simulink model "qdrdacsim"  (R2012b)
(part 2 of 52)

  zero_bool_3 : xbsIndex_r4/Constant  const=1  gui_display_data_type=Boolean  arith_type=Boolean  n_bits=36  bin_pt=0  preci_type=Single  exp_width=8  frac_width=24  explicit_period=on  period=1  equ=P=C  opselect=C  inp2=PCIN>>17  opr=+  inp1=P  carry=CIN  dbl_ovrd=off  block_type=constant
  zero_bool_7 : xbsIndex_r4/Constant  const=0  gui_display_data_type=Boolean  arith_type=Boolean  n_bits=36  bin_pt=0  preci_type=Single  exp_width=8  frac_width=24  explicit_period=on  period=1  equ=P=C  opselect=C  inp2=PCIN>>17  opr=+  inp1=P  carry=CIN  dbl_ovrd=off  block_type=constant
  wires:
  SRAM_LUT/9(syncout) -> Delay30/1
  MKID_ADC/9(sync) -> Delay29/1
  bool/1 -> octoscope/11(tr2), octoscope/12(tr3), octoscope/16(we3), octoscope/13(we0), octoscope/15(we2), octoscope/14(we1)
  ModSinNoise/1(I0) -> Delay21/1
  ModSinNoise/2(I1) -> Delay22/1
  ModSinNoise/3(I2) -> Delay23/1
  ModSinNoise/4(I3) -> Delay24/1
  ModSinNoise/5(Q0) -> Delay25/1
  ModSinNoise/6(Q1) -> Delay26/1
  ModSinNoise/7(Q2) -> Delay27/1
  ModSinNoise/8(Q3) -> Delay28/1
  SRAM_LUT/10(bus128) -> Delay36/1, Delay8/1
  Delay25/1 -> ri_to_c/2, octoscope/5(in5)
  Delay21/1 -> ri_to_c/1, octoscope/1(In1)
  Delay22/1 -> ri_to_c1/1, octoscope/2(In2)
  Delay26/1 -> ri_to_c1/2, octoscope/6(in6)
  Delay23/1 -> ri_to_c2/1, octoscope/3(In3)
  Delay27/1 -> ri_to_c2/2, octoscope/7(in7)
  Delay24/1 -> ri_to_c3/1, octoscope/4(In4)
  Delay28/1 -> ri_to_c3/2, octoscope/8(in8)
  fftcoefselector/2(we0) -> rect2polarV5/1(dvalid)
  fftcoefselector/3(we1) -> rect2polarV1/1(dvalid)
  fftcoefselector/4(we2) -> rect2polarV2/1(dvalid)
  fftcoefselector/5(we3) -> rect2polarV3/1(dvalid)
  fftcoefselector/6(chan0) -> rect2polarV5/3(chan)
  fftcoefselector/7(chan1) -> rect2polarV1/3(chan)
  fftcoefselector/8(chan2) -> rect2polarV2/3(chan)
  fftcoefselector/9(chan3) -> rect2polarV3/3(chan)
  Delay/1 -> rect2polarV5/2(cmplx)
  Delay1/1 -> rect2polarV1/2(cmplx)
  Delay2/1 -> rect2polarV2/2(cmplx)
  Delay3/1 -> rect2polarV3/2(cmplx)
  zero_bool_3/1 -> FIFO64_4/8, FIFO64_4/7, FIFO64_2/7, FIFO64_2/8, FIFO64_1/7, FIFO64_1/8, FIFO64_3/7, FIFO64_3/8
  FIFO64_4/1 -> Gateway Out33/1, sync_bit3/1, datamux/2
  FIFO64_4/2 -> emptymux/2
  FIFO64_4/3 -> quartfull/2
  FIFO64_4/8 -> Gateway Out34/1, vldmux/2
  lsb0_5_1/1 -> [rdchan_a]
  [rdchan_a] -> FIFO64_4/4
  [muxsel_a] -> Delay18/1
  Delay18/1 -> vldmux/1, quartfull/1, emptymux/1, datamux/1
  emptymux/1 -> MCode/2
  quartfull/1 -> MCode/3
  vldmux/1 -> Delay20/1
  fifoRdSettingsA/1(Out1) -> MCode/1, [dumpfifo]
  fifoRdSettingsA/3(Out3) -> [wrrawdata]
  fifoRdSettingsA/4(Out4) -> MCode/11, [is_look_sync]
  fifoRdSettingsA/5(Out5) -> MCode/8, [flushfifo]
  Constant/1 -> lastReadChanA/1(sim_1)
  fifoRdSettingsA/6(Out6) -> [fiforst]
  [fiforst] -> FIFO64_4/6
  Logical10/1 -> [fiford0]
  Logical11/1 -> [fiford1]
  Inverter/1 -> Logical10/1
  bits6_/1 -> Logical11/2, Inverter/1, [muxsel_a]
  MCode/1 -> Gateway Out16/1, Logical11/1, Logical10/2
  [fiford0] -> FIFO64_4/5
  PhaseCorrect1/2(cmplx_dout) -> c_to_ri5/1, dataformatter2/3(data)
  PhaseCorrect1/4(sync_out) -> Gateway Out21/1
  rect2polarV1/3(chandly) -> FIFO64_2/1
  [rdchan_a] -> FIFO64_2/4
  [fiford1] -> FIFO64_2/5
  [fiforst] -> FIFO64_2/6
  FIFO64_2/3 -> quartfull/3
  FIFO64_2/2 -> emptymux/3
  FIFO64_2/1 -> Gateway Out35/1, sync_bit4/1, datamux/3
  FIFO64_2/8 -> Gateway Out36/1, vldmux/3
  rect2polarV5/2(pol) -> scope_a2/1(In1), Concat3/2
  rect2polarV1/2(pol) -> scope_a2/2(In2), Concat2/2
  rect2polarV5/3(chandly) -> FIFO64_4/1
  fftcoefselector/11(fftfoecsync) -> Delay35/1, [fft_coef_sync]
  zero_bool_7/1 -> octoscope1/15(we2), octoscope1/14(we1), octoscope1/13(we0), octoscope1/12(tr3), octoscope1/10(tr1), octoscope1/11(tr2), octoscope1/16(we3)
  fifoRdSettingsA/7(Out7) -> [drop_all_events]
  Constant1/1 -> txdestport/1(sim_1), txdestip/1(sim_1)
  txdestip/1(in_reg) -> Delay12/1
  txdestport/1(in_reg) -> Delay13/1
  Concat1/1 -> Delay9/1
  fifoRdSettingsA/8(Out8) -> [ethernet_rst]
  bool_1/1 -> xmit0/8, xmit0/7
  xmit0/1 -> Delay15/1
  xmit0/3 -> Delay16/1
  xmit0/4 -> Delay17/1
  xmit0/5 -> Delay19/1
  rect2polarV2/2(pol) -> scope_a2/3(In3), Concat4/2
  rect2polarV3/2(pol) -> scope_a2/4(In4), Concat/2
  rect2polarV2/3(chandly) -> FIFO64_1/1
  rect2polarV3/3(chandly) -> FIFO64_3/1
  [fiforst] -> FIFO64_1/6
  [fiforst] -> FIFO64_3/6
  [dumpfifo] -> MCode2/1
  FIFO64_1/1 -> Gateway Out55/1, datamux1/2, sync_bit5/1
  FIFO64_1/2 -> emptymux1/2
  FIFO64_3/2 -> emptymux1/3
  FIFO64_1/3 -> quartfull1/2
  FIFO64_3/3 -> quartfull1/3
  FIFO64_1/8 -> Gateway Out56/1, vldmux1/2
  FIFO64_3/8 -> Gateway Out58/1, vldmux1/3
  Delay5/1 -> vldmux1/1, quartfull1/1, emptymux1/1, datamux1/1
  lsb0_5_2/1 -> [rdchan_b]
  Logical1/1 -> [fiford2]
  Logical3/1 -> [fiford3]
  Inverter1/1 -> Logical1/1
  bits6_1/1 -> Inverter1/1, Logical3/1, [muxsel_b]
  MCode2/1 -> Logical3/2, Logical1/2
  emptymux1/1 -> MCode2/2
  quartfull1/1 -> MCode2/3
  vldmux1/1 -> Delay6/1
  [muxsel_b] -> Delay5/1
  [rdchan_b] -> FIFO64_3/4
  [rdchan_b] -> FIFO64_1/4
  [fiford2] -> FIFO64_1/5
  [fiford3] -> FIFO64_3/5
  datamux1/1 -> PhaseCorrect2/2(cmplx_din), sync_bit1/1
  dataformatter1/1(dout) -> SinglaEvtFIFO2/1
  MCode4/5 -> Counter12/2, Delay10/1
  Inverter2/1 -> Gateway Out49/1, MCode4/1
  [fsmrst] -> MCode4/3
  MCode4/2 -> Counter16/2, Gateway Out64/1, OutFIFO1/3
  0xffffffff/1 -> quartfull2/5, quartfull3/5, quartfull3/2, quartfull2/2
  OutFIFO1/1 -> Gateway Out63/1, quartfull3/4
  OutFIFO1/4 -> Inverter3/1
  OutFIFO/1 -> Gateway Out65/1, quartfull2/4
  MCode4/3 -> Gateway Out47/1, quartfull2/1
  MCode4/4 -> Gateway Out48/1, quartfull3/1
  quartfull2/1 -> Concat1/1
  quartfull3/1 -> Concat1/2
  MCode4/1 -> Counter17/2, Gateway Out66/1, OutFIFO/3
  Delay8/1 -> MKID_DAC/1(buss128)
  Delay9/1 -> Slice1/1, Slice/1, xmit0/2
  Delay10/1 -> Gateway Out52/1, xmit0/3
  Delay11/1 -> Gateway Out53/1, xmit0/6
  Delay12/1 -> xmit0/4
  Delay13/1 -> xmit0/5
  [ethernet_rst] -> Delay14/1
  Delay14/1 -> xmit0/1
  Delay19/1 -> Counter11/2
  Delay29/1 -> octoscope/9(tr0)
  Delay30/1 -> fftcoefselector/2(lut_sync), octoscope/10(tr1)
  OutFIFO/4 -> Inverter2/1
  Inverter3/1 -> Gateway Out54/1, MCode4/2
  fifoRdSettingsA/9(Out9) -> [rst_full_counters]
  rect2polarV5/1(dvalidout) -> FIFO64_4/2, Counter2/2
  [rst_full_counters] -> Counter2/1
  Counter2/1 -> fifowrA/1(out_reg)
  Counter3/1 -> fifowriB/1(out_reg)
  [rst_full_counters] -> Counter3/1
  rect2polarV1/1(dvalidout) -> Counter3/2, FIFO64_2/2
  Counter4/1 -> fifowrC/1(out_reg)
  [rst_full_counters] -> Counter4/1
  rect2polarV2/1(dvalidout) -> Counter4/2, FIFO64_1/2
  Counter5/1 -> fifowrD/1(out_reg)
  [rst_full_counters] -> Counter5/1
  rect2polarV3/1(dvalidout) -> Counter5/2, FIFO64_3/2, scope_a2/5(sync)
  Counter6/1 -> evtfifowrA/1(out_reg)
  Counter7/1 -> evtfifowrB/1(out_reg)
  [rst_full_counters] -> Counter7/1
  Counter8/1 -> outfifowrA/1(out_reg)
  [rst_full_counters] -> Counter8/1
  Counter9/1 -> outfifowrB/1(out_reg)
  [rst_full_counters] -> Counter9/1
  [rst_full_counters] -> Counter10/1
  MCode4/6 -> Counter10/2, Counter12/1, Delay11/1
  Counter11/1 -> gbtxovfcnt/1(out_reg)
  Counter12/1 -> gbdatalen/1(out_reg)
  [rst_full_counters] -> Counter11/1
  Counter10/1 -> quartfull2/3, quartfull3/3, gbeofcount/1(out_reg)
  datamux/1 -> sync_bit/1, PhaseCorrect1/2(cmplx_din)
  [datapath_enable] -> Gateway Out23/1, PhaseCorrect1/4(en)
  Delay20/1 -> Gateway Out26/1, PhaseCorrect1/1(dvld_in)
  [datapath_enableb] -> PhaseCorrect2/4(en)
  PhaseCorrect2/2(cmplx_dout) -> dataformatter1/3(data)
  Delay6/1 -> PhaseCorrect2/1(dvld_in)
  [flushfifo] -> MCode4/4
  c_to_ri3/1 -> top16_8/1
  c_to_ri4/1 -> top16_2/1
  c_to_ri1/1 -> Gateway Out3/1, top16_3/1
  c_to_ri3/2 -> top16_5/1
  c_to_ri4/2 -> top16_6/1
  c_to_ri1/2 -> Gateway Out8/1, top16_7/1
  Delay35/1 -> octoscope1/9(tr0)
  Delay31/1 -> c_to_ri2/1
  Delay32/1 -> c_to_ri3/1
  Delay33/1 -> c_to_ri4/1
  Delay34/1 -> c_to_ri1/1
  top16_2/1 -> octoscope1/3(In3)
  top16_3/1 -> octoscope1/4(In4)
  top16_4/1 -> Gateway Out7/1, uint16_1/1, octoscope1/5(in5)
  top16_5/1 -> octoscope1/6(in6)
  top16_6/1 -> octoscope1/7(in7)
  top16_7/1 -> octoscope1/8(in8)
  Delay36/1 -> MKID_ADC/1(in128)
  Delay40/1 -> FFT512_/5(pol3)
  pfb_fir1/5(pol1_out4) -> scope_a/4(In4), Delay40/1
  pfb_fir1/4(pol1_out3) -> scope_a/3(In3), Delay39/1
  pfb_fir1/3(pol1_out2) -> scope_a/2(In2), Delay38/1
  Delay38/1 -> FFT512_/2(pol1)
  pfb_fir1/2(pol1_out1) -> scope_a/1(In1), Delay37/1
  Delay39/1 -> FFT512_/4(pol2)
  Delay41/1 -> Gateway Out9/1, FFT512_/3(syncin)
  Delay37/1 -> FFT512_/1(pol0)
  FFT512_/1(polo0) -> scope_a1/1(In1), Delay/1, Delay31/1
  FFT512_/3(polo1) -> scope_a1/2(In2), Delay32/1, Delay1/1
  FFT512_/4(polo2) -> scope_a1/3(In3), Delay33/1, Delay2/1
  FFT512_/5(polo3) -> scope_a1/4(In4), Delay34/1, Delay3/1
  FFT512_/2(sincout) -> Gateway Out10/1, scope_a1/5(sync), fftcoefselector/1(fftsyncout)
  fftcoefselector/13(topfbsyncin) -> pfb_fir1/1(sync), Gateway Out11/1
  ri_to_c/1 -> pfb_fir1/2(pol1_in1)
  ri_to_c1/1 -> pfb_fir1/3(pol1_in2)
  ri_to_c2/1 -> pfb_fir1/4(pol1_in3)
  ri_to_c3/1 -> pfb_fir1/5(pol1_in4)
  Gateway Out7/1 -> pfbscope/4
  Gateway Out4/1 -> pfbscope/1
  Gateway Out2/1 -> pfbscope/6
  Gateway Out6/1 -> pfbscope/3
  Gateway Out3/1 -> pfbscope/7
  Gateway Out8/1 -> pfbscope/8
  Gateway Out5/1 -> pfbscope/2
  Gateway Out1/1 -> pfbscope/5
  c_to_ri2/1 -> top16_1/1, Gateway Out4/1
  c_to_ri2/2 -> Gateway Out5/1, top16_4/1
  top16_1/1 -> uint16_0/1, Gateway Out6/1, octoscope1/1(In1)
  top16_8/1 -> octoscope1/2(In2)
  uint16_0/1 -> Gateway Out1/1
  uint16_1/1 -> Gateway Out2/1
  pfb_fir1/1(sync_out) -> Delay41/1, scope_a/5(sync)
  Gateway Out9/1 -> syncsc/1
  Gateway Out10/1 -> syncsc/2
  fftcoefselector/15(stopfft) -> Gateway Out12/1, FFT512_/6(rstn)
  Gateway Out11/1 -> syncsc/3
  Gateway Out12/1 -> syncsc/4
  fftcoefselector/12(fftshiftx) -> FFT512_/7(shift)
  catch_sync/1 -> Logical5/1, out5/1, align_sync_to_fft/1
  [fft_coef_sync] -> Logical/2, out3/1, align_sync_to_fft/2
  Logical/1 -> out4/1, catch_sync/2
  Inverter4/1 -> Logical/1
  Concat/1 -> FIFO64_3/3
  Concat4/1 -> FIFO64_1/3
  Concat2/1 -> FIFO64_2/3
  Concat3/1 -> sync_bit2/1, FIFO64_4/3
  [is_look_sync] -> dataformatter1/4(is_pulse)
  [is_look_sync] -> dataformatter2/4(is_pulse)
  count_16bit_/1 -> Relational/1, Relational1/1
  Relational1/1 -> count_16bit_/2
  Constant4/1 -> Relational1/2
  syncDelay/1(in_reg) -> Relational/2
  edge_detect/1(out) -> Counter1/2, out1/1, count_16bit_/1
  Relational/1 -> out2/1, Logical5/2, Inverter4/1
  Gateway Out/1 -> Display/1
  FIFO64_3/9 -> Gateway Out/1
  Constant5/1 -> syncDelay/1(sim_1)
  Pulse Generator/1 -> sync_in/1
  out7/1 -> Scope1/1
  out1/1 -> Scope1/2
  out2/1 -> Scope1/3
  out3/1 -> Scope1/4
  out4/1 -> Scope1/5
  out5/1 -> Scope1/6
  Logical5/1 -> catch_sync/1
  MCode/3 -> Gateway Out18/1, lsb0_5_1/1, bits6_/1, roachscope/2(In2), dataformatter2/2(channel_), Gateway Out27/1, PhaseCorrect1/3(chan)
  MCode/7 -> Gateway Out14/1, Counter15/2, Gateway Out15/1, [save_event]
  MCode/5 -> [datapath_enable]
  fifoRdSettingsA/2(Out2) -> MCode/4, [fsmrst]
  lastReadChanA/1(in_reg) -> MCode2/6, MCode/6
  readFifoSize/1(in_reg) -> [event_length], MCode2/9, MCode/9
  Constant6/1 -> readFifoSize/1(sim_1)
  PhaseCorrect1/1(dvld_out) -> MCode/5, MCode/12, Gateway Out24/1
  [fsmrst] -> MCode2/4
  MCode2/3 -> dataformatter1/2(channel_), PhaseCorrect2/3(chan), lsb0_5_2/1, bits6_1/1
  MCode2/5 -> [datapath_enableb]
  PhaseCorrect2/1(dvld_out) -> MCode2/5
  MCode2/7 -> FRD1/4(new_evt_rdy), Counter14/2
  [flushfifo] -> MCode2/8
  [is_look_sync] -> MCode2/11
  bool_4/1 -> MCode/7
  bool_5/1 -> MCode2/7
  bool_6/1 -> MCode2/12
  MCode/9 -> Gateway Out20/1
  Gateway Out19/1 -> fifofsmscope/4
  Gateway Out16/1 -> fifofsmscope/1
  Gateway Out14/1 -> fifofsmscope/6
  Gateway Out18/1 -> fifofsmscope/3
  Gateway Out15/1 -> fifofsmscope/7
  Gateway Out20/1 -> fifofsmscope/8
  Gateway Out17/1 -> fifofsmscope/2
  Gateway Out13/1 -> fifofsmscope/5
  MCode/4 -> Gateway Out28/1, Gateway Out19/1
  Gateway Out27/1 -> phasecorrectscope/4
  Gateway Out24/1 -> phasecorrectscope/1
  Gateway Out22/1 -> phasecorrectscope/6
  Gateway Out26/1 -> phasecorrectscope/3
  Gateway Out23/1 -> phasecorrectscope/7
  Gateway Out28/1 -> phasecorrectscope/8
  Gateway Out25/1 -> phasecorrectscope/2
  Gateway Out21/1 -> phasecorrectscope/5
  Delay42/1 -> Gateway Out22/1, MCode/10
  c_to_ri5/1 -> Gateway Out25/1
  sync_bit/1 -> Delay42/1
  sync_bit1/1 -> Delay43/1
  Delay43/1 -> MCode2/10
  dataformatter2/1(dout) -> Gateway Out37/1, SinglaEvtFIFO1/1
  Counter1/1 -> numSyncPulses/1(out_reg)
  [rst_full_counters] -> Counter1/1
  Counter13/1 -> numSyncPulses1/1(out_reg)
  [rst_full_counters] -> Counter13/1
  Mux/1 -> edge_detect/1(in)
  sync_in/1 -> Mux/2
  fifoRdSettingsA/10(Out10) -> [sync_source]
  [sync_source] -> Mux/1
  RampGenerator/1(ramp) -> SigmaDeltaSecOrder/1(DataIn)
  RampGenerator/2(syncout) -> Mux/3
  Constant2/1 -> sw_timestamp2/1(sim_1)
  align_sync_to_fft/1 -> Counter13/2, out7/1, Concat5/2
  sw_timestamp2/1(in_reg) -> low2bits_/1
  low2bits_/1 -> Concat5/1
  fftcoefselector/17(timestamp) -> [fftcounter]
  PhaseCorrect1/5(swts) -> roachscope/1(In1)
  PhaseCorrect2/5(swts) -> Gateway Out43/1
  sw_timestamp/1(in_reg) -> dataformatter1/1(timestamp32_), dataformatter2/1(timestamp32_)
  Gateway Out38/1 -> wrsingevt/2
  Gateway Out37/1 -> wrsingevt/1
  Gateway Out39/1 -> sync_ts1/1
  Gateway Out40/1 -> sync_ts1/2
  Gateway Out42/1 -> sync_ts1/3
  sync_bit3/1 -> roachscope/5(In5), Gateway Out42/1
  Gateway Out43/1 -> sync_ts2/2
  Gateway Out41/1 -> sync_ts2/1
  PhaseCorrect2/4(sync_out) -> Gateway Out41/1
  sync_bit4/1 -> roachscope/6(In6), Gateway Out44/1
  Gateway Out44/1 -> sync_ts1/4
  sync_bit5/1 -> roachscope/7(In7), Gateway Out45/1
  Gateway Out45/1 -> sync_ts1/5
  Gateway Out46/1 -> sync_ts1/6
  FIFO64_3/1 -> Gateway Out57/1, sync_bit6/1, datamux1/3
  Concat5/1 -> Concat2/1, roachscope/3(In3), Gateway Out39/1, Concat3/1, Concat4/1, Concat/1
  sync_bit2/1 -> roachscope/4(In4), Gateway Out40/1
  sync_bit6/1 -> roachscope/8(In8), Gateway Out46/1
  Counter14/1 -> numdoneevts1/1(out_reg)
  [rst_full_counters] -> Counter14/1
  Counter15/1 -> numdoneevts0/1(out_reg)
  [rst_full_counters] -> Counter15/1
  Counter16/1 -> outfifordB/1(out_reg)
  [rst_full_counters] -> Counter16/1
  Counter17/1 -> outfifordA/1(out_reg)
  [rst_full_counters] -> Counter17/1
  Counter18/1 -> evtfifordA/1(out_reg)
  [rst_full_counters] -> Counter18/1, Counter6/1
  Counter19/1 -> evtfifordB/1(out_reg)
  [rst_full_counters] -> Counter19/1
  Constant3/1 -> sw_timestamp/1(sim_1)
  Gateway Out53/1 -> outfifogbtx/4
  Gateway Out50/1 -> outfifogbtx/1
  Gateway Out48/1 -> outfifogbtx/6
  Gateway Out52/1 -> outfifogbtx/3
  Gateway Out49/1 -> outfifogbtx/7
  Gateway Out54/1 -> outfifogbtx/8
  Gateway Out51/1 -> outfifogbtx/2
  Gateway Out47/1 -> outfifogbtx/5
  Slice/1 -> Gateway Out50/1
  Slice1/1 -> Gateway Out51/1
  SigmaDeltaSecOrder/1(DataOut) -> Delay4/1
  Delay4/1 -> sync_out/1
  fifoRdSettingsA/11(Out11) -> [en_ramp_gen]
  [en_ramp_gen] -> Delay4/2
  MCode/6 -> dataformatter2/5(wr_data_sel), Gateway Out13/1
  MCode2/6 -> dataformatter1/5(wr_data_sel)
  MCode2/2 -> Counter7/2, SinglaEvtFIFO2/2
  MCode/2 -> Gateway Out17/1, Counter6/2, Gateway Out38/1, SinglaEvtFIFO1/2
  [flushfifo] -> FRD/6(clr_fifos)
  [fsmrst] -> FRD/5(rst)
  [event_length] -> FRD/1(evtlen)
  SinglaEvtFIFO1/2 -> FRD/2(fifo_empty)
  SinglaEvtFIFO1/1 -> Gateway Out29/1, FRD/3(data_in)
  [save_event] -> FRD/4(new_evt_rdy)
  FRD/2(dataout) -> Gateway Out31/1, OutFIFO/1
  FRD/3(out_wr) -> Counter8/2, Gateway Out32/1, OutFIFO/2
  FRD/1(evt_fifo_rd) -> Counter18/2, Gateway Out30/1, SinglaEvtFIFO1/3
  fifoRdSettingsA/12(Out12) -> [fluxdemod]
  fifoRdSettingsA/13(Out13) -> [savefluxraw]
  [savefluxraw] -> FRD/8(savefluxraw)
  [fluxdemod] -> FRD/7(isflux_demod)
  [fsmrst] -> FRD1/5(rst)
  [flushfifo] -> FRD1/6(clr_fifos)
  SinglaEvtFIFO2/1 -> FRD1/3(data_in), Gateway Out59/1
  FRD1/2(dataout) -> OutFIFO1/1, Gateway Out61/1
  FRD1/1(evt_fifo_rd) -> Gateway Out60/1, Counter19/2, SinglaEvtFIFO2/3
  SinglaEvtFIFO2/2 -> FRD1/2(fifo_empty)
  [event_length] -> FRD1/1(evtlen)
  [fluxdemod] -> FRD1/7(isflux_demod)
  [savefluxraw] -> FRD1/8(savefluxraw)
  FRD1/3(out_wr) -> Gateway Out62/1, OutFIFO1/2, Counter9/2
  Gateway Out30/1 -> rdsingevt/2
  Gateway Out29/1 -> rdsingevt/1
  Gateway Out32/1 -> wroutfifo/2
  Gateway Out31/1 -> wroutfifo/1
  Gateway Out34/1 -> sync_ts3/2
  Gateway Out33/1 -> sync_ts3/1
  Gateway Out36/1 -> sync_ts4/2
  Gateway Out35/1 -> sync_ts4/1
  Gateway Out56/1 -> sync_ts5/2
  Gateway Out55/1 -> sync_ts5/1
  Gateway Out58/1 -> sync_ts6/2
  Gateway Out57/1 -> sync_ts6/1
  Gateway Out60/1 -> rdsingevt1/2
  Gateway Out59/1 -> rdsingevt1/1
  Gateway Out62/1 -> wroutfifo2/2
  Gateway Out61/1 -> wroutfifo2/1
  Gateway Out64/1 -> rdoutfifo2/2
  Gateway Out63/1 -> rdoutfifo2/1
  Gateway Out66/1 -> rdoutfifo1/2
  Gateway Out65/1 -> rdoutfifo1/1
